simulink model "seven_segment_display"  (R2023b)
settings: Solver=VariableStepAuto  StartTime=0.0  StopTime=inf  RelTol=1e-3
libraries: simulink_extras x33
settings Model: ModifiedByFormat=ayber  Creator=ayber  LastModifiedBy=ayber
settings OptimizationCC: ReuseModelBlockBuffer=off

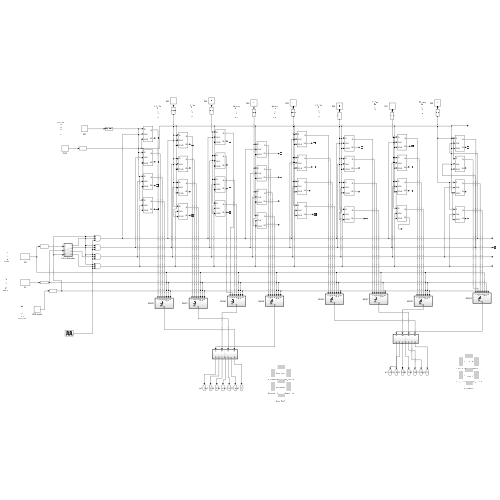
[thumbnail: Simulink's stored preview of the top-level diagram]
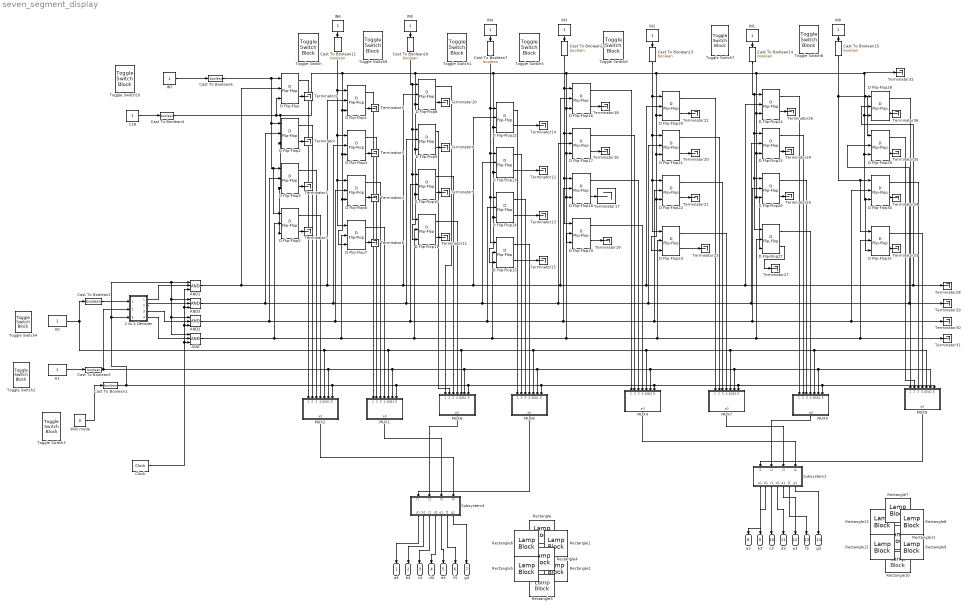
== system seven_segment_display ==
  2 to 4 Decoder : Subsystem  TreatAsAtomicUnit=on
  A0 : Constant
  A1 : Constant
  AND{,1..3} (4 alike) : Logic  Inputs=3  IconShape=distinctive  AllPortsSameDT=off  OutDataTypeStr=boolean
  CLR : Constant
  Cast To Boolean{1..2,4..7,10..15} (12 alike) : DataTypeConversion  OutDataTypeStr=boolean  SaturateOnIntegerOverflow=off  RndMeth=Floor
  Clock : simulink_extras/Flip Flops/Clock  period=2
  D Flip-Flop{,1..31} (32 alike) : simulink_extras/Flip Flops/D Flip-Flop
  IN{0..7} (8 alike) : Constant
  MUX1 : Subsystem  TreatAsAtomicUnit=on
  MUX2 : Subsystem  TreatAsAtomicUnit=on
  MUX4 : Subsystem  TreatAsAtomicUnit=on
  MUX5 : Subsystem  TreatAsAtomicUnit=on
  MUX6 : Subsystem  TreatAsAtomicUnit=on
  MUX7 : Subsystem  TreatAsAtomicUnit=on
  MUX8 : Subsystem  TreatAsAtomicUnit=on
  MUX9 : Subsystem  TreatAsAtomicUnit=on
  Rectangle{,1..13} (14 alike) : LampBlock  LabelPosition=Bottom  Icon=Rectangle
  Subsystem1 : Subsystem  TreatAsAtomicUnit=on
  Subsystem4 : Subsystem  TreatAsAtomicUnit=on
  Terminator{,1..36} (37 alike) : Terminator
  Toggle Switch{,1,5..10} (8 alike) : ToggleSwitchBlock
      settings: Values={{'Off', 'On'}, [0 1]}
  Toggle Switch2 : ToggleSwitchBlock  LabelPosition=Bottom
      settings: Values={{'Off', 'On'}, [0 1]}
  Toggle Switch3 : ToggleSwitchBlock  LabelPosition=Bottom
      settings: Values={{'Off', 'On'}, [0 1]}
  Toggle Switch4 : ToggleSwitchBlock  LabelPosition=Bottom
      settings: Values={{'Off', 'On'}, [0 1]}
  W/R mode : Constant  Value=0
  a4 : Outport
  b4 : Outport  Port=2
  c4 : Outport  Port=3
  d4 : Outport  Port=4
  e4 : Outport  Port=5
  f4 : Outport  Port=6
  g4 : Outport  Port=7
  a3 : Outport  Port=8
  b3 : Outport  Port=9
  c3 : Outport  Port=10
  d3 : Outport  Port=11
  e3 : Outport  Port=12
  f3 : Outport  Port=13
  g3 : Outport  Port=14
  wires:
  D Flip-Flop2/2 -> Terminator/1
  D Flip-Flop3/2 -> Terminator1/1
  CLR/1 -> Cast To Boolean4/1
  W/R mode/1 -> Cast To Boolean1/1
  A0/1 -> MUX9/5(A0), MUX5/5(A0), MUX7/5(A0), MUX4/5(A0), MUX8/5(A0), MUX6/5(A0), MUX1/5(A0), MUX2/5(A0), Cast To Boolean2/1
  A1/1 -> Cast To Boolean5/1
  D Flip-Flop/2 -> Terminator2/1
  D Flip-Flop5/2 -> Terminator7/1
  D Flip-Flop1/2 -> Terminator5/1
  D Flip-Flop7/2 -> Terminator6/1
  D Flip-Flop6/2 -> Terminator4/1
  D Flip-Flop4/2 -> Terminator3/1
  D Flip-Flop8/2 -> Terminator10/1
  D Flip-Flop11/2 -> Terminator11/1
  D Flip-Flop10/2 -> Terminator9/1
  D Flip-Flop9/2 -> Terminator8/1
  D Flip-Flop12/2 -> Terminator14/1
  D Flip-Flop15/2 -> Terminator15/1
  D Flip-Flop14/2 -> Terminator13/1
  D Flip-Flop13/2 -> Terminator12/1
  D Flip-Flop19/2 -> Terminator19/1
  D Flip-Flop18/2 -> Terminator17/1
  D Flip-Flop17/2 -> Terminator16/1
  D Flip-Flop16/2 -> Terminator18/1
  D Flip-Flop23/2 -> Terminator23/1
  D Flip-Flop22/2 -> Terminator21/1
  D Flip-Flop21/2 -> Terminator20/1
  D Flip-Flop20/2 -> Terminator22/1
  IN7/1 -> Cast To Boolean6/1
  Cast To Boolean6/1 -> D Flip-Flop/1, D Flip-Flop5/1, D Flip-Flop3/1, D Flip-Flop2/1
  IN4/1 -> Cast To Boolean7/1
  Cast To Boolean7/1 -> D Flip-Flop15/1, D Flip-Flop14/1, D Flip-Flop13/1, D Flip-Flop12/1
  IN5/1 -> Cast To Boolean10/1
  Cast To Boolean10/1 -> D Flip-Flop9/1, D Flip-Flop11/1, D Flip-Flop10/1, D Flip-Flop8/1
  IN6/1 -> Cast To Boolean11/1
  IN3/1 -> Cast To Boolean12/1
  IN2/1 -> Cast To Boolean13/1
  IN1/1 -> Cast To Boolean14/1
  D Flip-Flop24/2 -> Terminator26/1
  D Flip-Flop26/2 -> Terminator25/1
  D Flip-Flop27/2 -> Terminator27/1
  D Flip-Flop25/2 -> Terminator24/1
  Cast To Boolean14/1 -> D Flip-Flop27/1, D Flip-Flop26/1, D Flip-Flop25/1, D Flip-Flop24/1
  Cast To Boolean13/1 -> D Flip-Flop22/1, D Flip-Flop23/1, D Flip-Flop21/1, D Flip-Flop20/1
  Cast To Boolean12/1 -> D Flip-Flop19/1, D Flip-Flop18/1, D Flip-Flop17/1, D Flip-Flop16/1
  Cast To Boolean11/1 -> D Flip-Flop4/1, D Flip-Flop6/1, D Flip-Flop7/1, D Flip-Flop1/1
  Cast To Boolean5/1 -> MUX2/6(A1), MUX1/6(A1), MUX6/6(A1), MUX8/6(A1), MUX4/6(A1), MUX7/6(A1), MUX5/6(A1), MUX9/6(A1), 2 to 4 Decoder/2(In2)
  Cast To Boolean2/1 -> 2 to 4 Decoder/1(In1)
  Clock/1 -> AND1/3, AND3/3, AND2/3, AND/3
  Cast To Boolean1/1 -> MUX9/7(E), MUX5/7(E), MUX7/7(E), MUX4/7(E), MUX8/7(E), MUX6/7(E), MUX1/7(E), MUX2/7(E), AND/1, AND2/1, AND3/1, AND1/1, 2 to 4 Decoder/3(E)
  2 to 4 Decoder/1(Out1) -> AND1/2
  2 to 4 Decoder/2(Out2) -> AND3/2
  2 to 4 Decoder/3(Out3) -> AND2/2
  2 to 4 Decoder/4(Out4) -> AND/2
  AND1/1 -> Terminator28/1, D Flip-Flop28/2, D Flip-Flop24/2, D Flip-Flop20/2, D Flip-Flop16/2, D Flip-Flop12/2, D Flip-Flop8/2, D Flip-Flop1/2, D Flip-Flop/2
  AND2/1 -> Terminator30/1, D Flip-Flop30/2, D Flip-Flop26/2, D Flip-Flop22/2, D Flip-Flop18/2, D Flip-Flop14/2, D Flip-Flop10/2, D Flip-Flop6/2, D Flip-Flop3/2
  AND3/1 -> D Flip-Flop29/2, Terminator29/1, D Flip-Flop25/2, D Flip-Flop21/2, D Flip-Flop17/2, D Flip-Flop13/2, D Flip-Flop9/2, D Flip-Flop4/2, D Flip-Flop2/2
  AND/1 -> Terminator31/1, D Flip-Flop31/2, D Flip-Flop27/2, D Flip-Flop23/2, D Flip-Flop19/2, D Flip-Flop15/2, D Flip-Flop11/2, D Flip-Flop7/2, D Flip-Flop5/2
  Cast To Boolean4/1 -> D Flip-Flop1/3, D Flip-Flop4/3, D Flip-Flop6/3, D Flip-Flop7/3, D Flip-Flop31/3, D Flip-Flop30/3, D Flip-Flop29/3, D Flip-Flop28/3, Terminator32/1, D Flip-Flop27/3, D Flip-Flop26/3, D Flip-Flop25/3, D Flip-Flop24/3, D Flip-Flop23/3, D Flip-Flop22/3, D Flip-Flop21/3, D Flip-Flop20/3, D Flip-Flop19/3, D Flip-Flop18/3, D Flip-Flop17/3, D Flip-Flop16/3, D Flip-Flop15/3, D Flip-Flop14/3, D Flip-Flop13/3, D Flip-Flop12/3, D Flip-Flop8/3, D Flip-Flop9/3, D Flip-Flop10/3, D Flip-Flop11/3, D Flip-Flop5/3, D Flip-Flop3/3, D Flip-Flop2/3, D Flip-Flop/3
  D Flip-Flop5/1 -> MUX2/4(In6)
  D Flip-Flop7/1 -> MUX1/4(In6)
  D Flip-Flop15/1 -> MUX8/4(In6)
  D Flip-Flop19/1 -> MUX4/4(In6)
  D Flip-Flop23/1 -> MUX7/4(In6)
  D Flip-Flop27/1 -> MUX5/4(In6)
  D Flip-Flop26/1 -> MUX5/3(In5)
  D Flip-Flop22/1 -> MUX7/3(In5)
  D Flip-Flop25/1 -> MUX5/2(In4)
  D Flip-Flop24/1 -> MUX5/1(In3)
  D Flip-Flop21/1 -> MUX7/2(In4)
  D Flip-Flop20/1 -> MUX7/1(In3)
  D Flip-Flop18/1 -> MUX4/3(In5)
  D Flip-Flop17/1 -> MUX4/2(In4)
  D Flip-Flop16/1 -> MUX4/1(In3)
  D Flip-Flop3/1 -> MUX2/3(In5)
  D Flip-Flop/1 -> MUX2/1(In3)
  D Flip-Flop2/1 -> MUX2/2(In4)
  D Flip-Flop1/1 -> MUX1/1(In3)
  D Flip-Flop4/1 -> MUX1/2(In4)
  D Flip-Flop6/1 -> MUX1/3(In5)
  D Flip-Flop8/1 -> MUX6/1(In3)
  D Flip-Flop9/1 -> MUX6/2(In4)
  D Flip-Flop10/1 -> MUX6/3(In5)
  D Flip-Flop11/1 -> MUX6/4(In6)
  D Flip-Flop12/1 -> MUX8/1(In3)
  D Flip-Flop13/1 -> MUX8/2(In4)
  D Flip-Flop14/1 -> MUX8/3(In5)
  D Flip-Flop31/2 -> Terminator33/1
  D Flip-Flop30/2 -> Terminator34/1
  D Flip-Flop29/2 -> Terminator35/1
  D Flip-Flop28/2 -> Terminator36/1
  D Flip-Flop28/1 -> MUX9/1(In3)
  D Flip-Flop29/1 -> MUX9/2(In4)
  D Flip-Flop30/1 -> MUX9/3(In5)
  D Flip-Flop31/1 -> MUX9/4(In6)
  IN0/1 -> Cast To Boolean15/1
  Cast To Boolean15/1 -> D Flip-Flop29/1, D Flip-Flop28/1, D Flip-Flop31/1, D Flip-Flop30/1
  Subsystem4/1(a1) -> a4/1
  Subsystem4/4(d1) -> d4/1
  Subsystem4/5(e1) -> e4/1
  Subsystem4/7(g1) -> g4/1
  Subsystem4/6(f1) -> f4/1
  Subsystem4/3(c1) -> c4/1
  Subsystem4/2(b1) -> b4/1
  MUX2/1(a0) -> Subsystem4/4(I4)
  MUX1/1(a0) -> Subsystem4/3(I3)
  MUX6/1(a0) -> Subsystem4/2(I2)
  MUX8/1(a0) -> Subsystem4/1(I1)
  Subsystem1/5(e1) -> e3/1
  Subsystem1/4(d1) -> d3/1
  Subsystem1/6(f1) -> f3/1
  Subsystem1/1(a1) -> a3/1
  Subsystem1/2(b1) -> b3/1
  Subsystem1/7(g1) -> g3/1
  Subsystem1/3(c1) -> c3/1
  MUX4/1(a0) -> Subsystem1/4(I4)
  MUX7/1(a0) -> Subsystem1/3(I3)
  MUX5/1(a0) -> Subsystem1/2(I2)
  MUX9/1(a0) -> Subsystem1/1(I1)

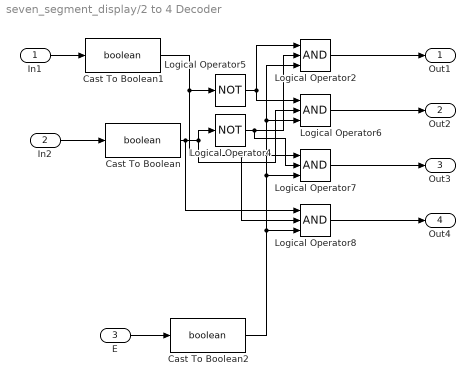
== system seven_segment_display/2 to 4 Decoder ==
  In1 : Inport
  In2 : Inport  Port=2
  E : Inport  Port=3
  Cast To Boolean : DataTypeConversion  OutDataTypeStr=boolean  SaturateOnIntegerOverflow=off  RndMeth=Floor
  Cast To Boolean1 : DataTypeConversion  OutDataTypeStr=boolean  SaturateOnIntegerOverflow=off  RndMeth=Floor
  Cast To Boolean2 : DataTypeConversion  OutDataTypeStr=boolean  SaturateOnIntegerOverflow=off  RndMeth=Floor
  Logical Operator{2,6..8} (4 alike) : Logic  Inputs=3  AllPortsSameDT=off  OutDataTypeStr=boolean
  Logical Operator4 : Logic  Operator=NOT  AllPortsSameDT=off  OutDataTypeStr=boolean
  Logical Operator5 : Logic  Operator=NOT  AllPortsSameDT=off  OutDataTypeStr=boolean
  Out1 : Outport
  Out2 : Outport  Port=2
  Out3 : Outport  Port=3
  Out4 : Outport  Port=4
  wires:
  Logical Operator8/1 -> Out4/1
  Logical Operator6/1 -> Out2/1
  Logical Operator2/1 -> Out1/1
  In1/1 -> Cast To Boolean1/1
  Cast To Boolean2/1 -> Logical Operator8/3, Logical Operator7/3, Logical Operator6/3, Logical Operator2/3
  Cast To Boolean/1 -> Logical Operator8/1, Logical Operator6/2, Logical Operator4/1
  Logical Operator7/1 -> Out3/1
  In2/1 -> Cast To Boolean/1
  Cast To Boolean1/1 -> Logical Operator8/2, Logical Operator7/1, Logical Operator5/1
  E/1 -> Cast To Boolean2/1
  Logical Operator5/1 -> Logical Operator6/1, Logical Operator2/1
  Logical Operator4/1 -> Logical Operator7/2, Logical Operator2/2

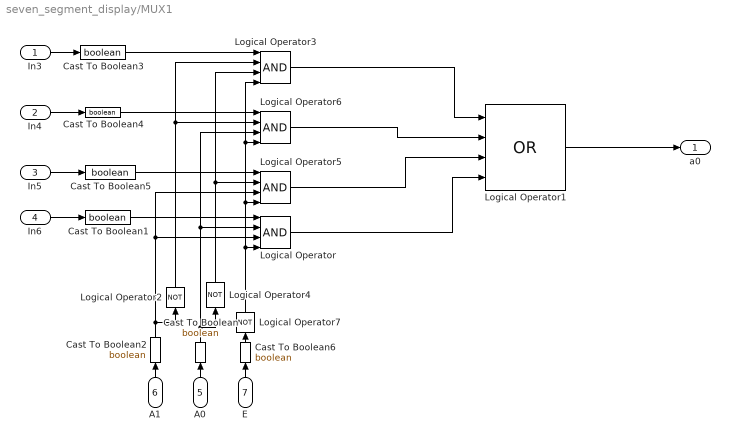
== system seven_segment_display/MUX1 ==
  In3 : Inport
  In4 : Inport  Port=2
  In5 : Inport  Port=3
  In6 : Inport  Port=4
  A0 : Inport  Port=5
  A1 : Inport  Port=6
  E : Inport  Port=7
  Cast To Boolean{,1..6} (7 alike) : DataTypeConversion  OutDataTypeStr=boolean  SaturateOnIntegerOverflow=off  RndMeth=Floor
  Logical Operator{,3,5..6} (4 alike) : Logic  Inputs=4  AllPortsSameDT=off  OutDataTypeStr=boolean
  Logical Operator1 : Logic  Operator=OR  Inputs=4  AllPortsSameDT=off  OutDataTypeStr=boolean
  Logical Operator2 : Logic  Operator=NOT  AllPortsSameDT=off  OutDataTypeStr=boolean
  Logical Operator4 : Logic  Operator=NOT  AllPortsSameDT=off  OutDataTypeStr=boolean
  Logical Operator7 : Logic  Operator=NOT  AllPortsSameDT=off  OutDataTypeStr=boolean
  a0 : Outport
  wires:
  A0/1 -> Cast To Boolean/1
  Logical Operator5/1 -> Logical Operator1/3
  In4/1 -> Cast To Boolean4/1
  Cast To Boolean3/1 -> Logical Operator3/1
  In5/1 -> Cast To Boolean5/1
  Cast To Boolean5/1 -> Logical Operator5/1
  Logical Operator1/1 -> a0/1
  Cast To Boolean1/1 -> Logical Operator/1
  Cast To Boolean4/1 -> Logical Operator6/1
  Logical Operator/1 -> Logical Operator1/4
  Logical Operator4/1 -> Logical Operator5/2, Logical Operator3/3
  In3/1 -> Cast To Boolean3/1
  Cast To Boolean/1 -> Logical Operator/2, Logical Operator6/3, Logical Operator4/1
  Logical Operator2/1 -> Logical Operator6/2, Logical Operator3/2
  A1/1 -> Cast To Boolean2/1
  In6/1 -> Cast To Boolean1/1
  Cast To Boolean2/1 -> Logical Operator/3, Logical Operator5/3, Logical Operator2/1
  Cast To Boolean6/1 -> Logical Operator7/1
  E/1 -> Cast To Boolean6/1
  Logical Operator7/1 -> Logical Operator3/4, Logical Operator6/4, Logical Operator5/4, Logical Operator/4
  Logical Operator6/1 -> Logical Operator1/2
  Logical Operator3/1 -> Logical Operator1/1

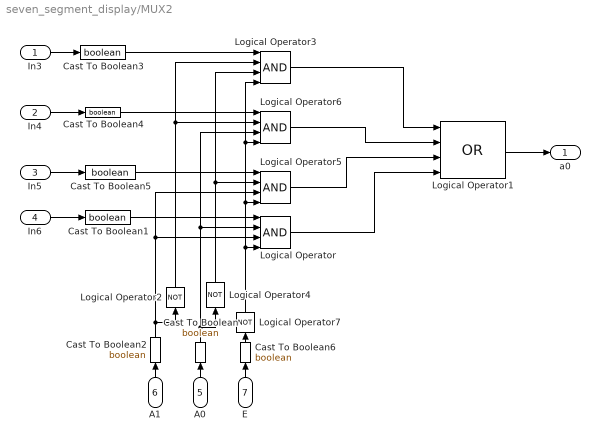
== system seven_segment_display/MUX2 ==
  In3 : Inport
  In4 : Inport  Port=2
  In5 : Inport  Port=3
  In6 : Inport  Port=4
  A0 : Inport  Port=5
  A1 : Inport  Port=6
  E : Inport  Port=7
  Cast To Boolean{,1..6} (7 alike) : DataTypeConversion  OutDataTypeStr=boolean  SaturateOnIntegerOverflow=off  RndMeth=Floor
  Logical Operator{,3,5..6} (4 alike) : Logic  Inputs=4  AllPortsSameDT=off  OutDataTypeStr=boolean
  Logical Operator1 : Logic  Operator=OR  Inputs=4  AllPortsSameDT=off  OutDataTypeStr=boolean
  Logical Operator2 : Logic  Operator=NOT  AllPortsSameDT=off  OutDataTypeStr=boolean
  Logical Operator4 : Logic  Operator=NOT  AllPortsSameDT=off  OutDataTypeStr=boolean
  Logical Operator7 : Logic  Operator=NOT  AllPortsSameDT=off  OutDataTypeStr=boolean
  a0 : Outport
  wires:
  A0/1 -> Cast To Boolean/1
  Logical Operator5/1 -> Logical Operator1/3
  In4/1 -> Cast To Boolean4/1
  Cast To Boolean3/1 -> Logical Operator3/1
  In5/1 -> Cast To Boolean5/1
  Cast To Boolean5/1 -> Logical Operator5/1
  Logical Operator1/1 -> a0/1
  Cast To Boolean1/1 -> Logical Operator/1
  Cast To Boolean4/1 -> Logical Operator6/1
  Logical Operator/1 -> Logical Operator1/4
  Logical Operator4/1 -> Logical Operator5/2, Logical Operator3/3
  In3/1 -> Cast To Boolean3/1
  Cast To Boolean/1 -> Logical Operator/2, Logical Operator6/3, Logical Operator4/1
  Logical Operator2/1 -> Logical Operator6/2, Logical Operator3/2
  A1/1 -> Cast To Boolean2/1
  In6/1 -> Cast To Boolean1/1
  Cast To Boolean2/1 -> Logical Operator/3, Logical Operator5/3, Logical Operator2/1
  Cast To Boolean6/1 -> Logical Operator7/1
  E/1 -> Cast To Boolean6/1
  Logical Operator7/1 -> Logical Operator3/4, Logical Operator6/4, Logical Operator5/4, Logical Operator/4
  Logical Operator6/1 -> Logical Operator1/2
  Logical Operator3/1 -> Logical Operator1/1

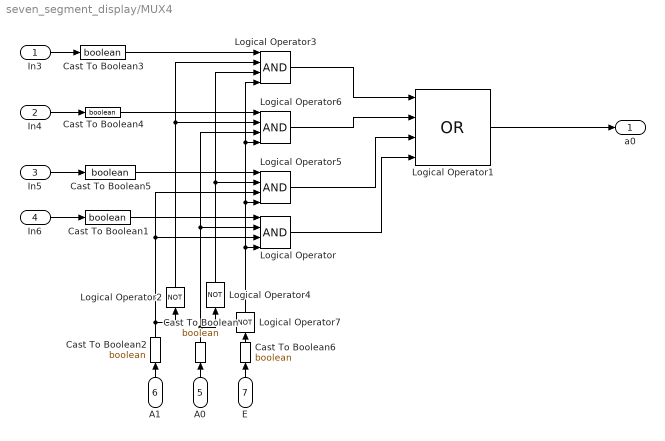
== system seven_segment_display/MUX4 ==
  In3 : Inport
  In4 : Inport  Port=2
  In5 : Inport  Port=3
  In6 : Inport  Port=4
  A0 : Inport  Port=5
  A1 : Inport  Port=6
  E : Inport  Port=7
  Cast To Boolean{,1..6} (7 alike) : DataTypeConversion  OutDataTypeStr=boolean  SaturateOnIntegerOverflow=off  RndMeth=Floor
  Logical Operator{,3,5..6} (4 alike) : Logic  Inputs=4  AllPortsSameDT=off  OutDataTypeStr=boolean
  Logical Operator1 : Logic  Operator=OR  Inputs=4  AllPortsSameDT=off  OutDataTypeStr=boolean
  Logical Operator2 : Logic  Operator=NOT  AllPortsSameDT=off  OutDataTypeStr=boolean
  Logical Operator4 : Logic  Operator=NOT  AllPortsSameDT=off  OutDataTypeStr=boolean
  Logical Operator7 : Logic  Operator=NOT  AllPortsSameDT=off  OutDataTypeStr=boolean
  a0 : Outport
  wires:
  A0/1 -> Cast To Boolean/1
  Logical Operator5/1 -> Logical Operator1/3
  In4/1 -> Cast To Boolean4/1
  Cast To Boolean3/1 -> Logical Operator3/1
  In5/1 -> Cast To Boolean5/1
  Cast To Boolean5/1 -> Logical Operator5/1
  Logical Operator1/1 -> a0/1
  Cast To Boolean1/1 -> Logical Operator/1
  Cast To Boolean4/1 -> Logical Operator6/1
  Logical Operator/1 -> Logical Operator1/4
  Logical Operator4/1 -> Logical Operator5/2, Logical Operator3/3
  In3/1 -> Cast To Boolean3/1
  Cast To Boolean/1 -> Logical Operator/2, Logical Operator6/3, Logical Operator4/1
  Logical Operator2/1 -> Logical Operator6/2, Logical Operator3/2
  A1/1 -> Cast To Boolean2/1
  In6/1 -> Cast To Boolean1/1
  Cast To Boolean2/1 -> Logical Operator/3, Logical Operator5/3, Logical Operator2/1
  Cast To Boolean6/1 -> Logical Operator7/1
  E/1 -> Cast To Boolean6/1
  Logical Operator7/1 -> Logical Operator3/4, Logical Operator6/4, Logical Operator5/4, Logical Operator/4
  Logical Operator3/1 -> Logical Operator1/1
  Logical Operator6/1 -> Logical Operator1/2

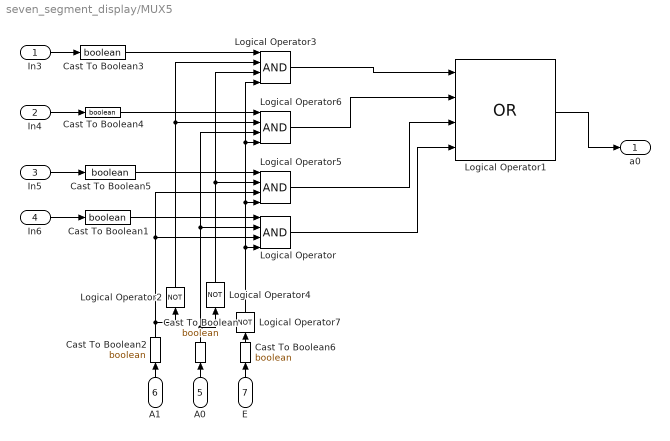
== system seven_segment_display/MUX5 ==
  In3 : Inport
  In4 : Inport  Port=2
  In5 : Inport  Port=3
  In6 : Inport  Port=4
  A0 : Inport  Port=5
  A1 : Inport  Port=6
  E : Inport  Port=7
  Cast To Boolean{,1..6} (7 alike) : DataTypeConversion  OutDataTypeStr=boolean  SaturateOnIntegerOverflow=off  RndMeth=Floor
  Logical Operator{,3,5..6} (4 alike) : Logic  Inputs=4  AllPortsSameDT=off  OutDataTypeStr=boolean
  Logical Operator1 : Logic  Operator=OR  Inputs=4  AllPortsSameDT=off  OutDataTypeStr=boolean
  Logical Operator2 : Logic  Operator=NOT  AllPortsSameDT=off  OutDataTypeStr=boolean
  Logical Operator4 : Logic  Operator=NOT  AllPortsSameDT=off  OutDataTypeStr=boolean
  Logical Operator7 : Logic  Operator=NOT  AllPortsSameDT=off  OutDataTypeStr=boolean
  a0 : Outport
  wires:
  A0/1 -> Cast To Boolean/1
  Logical Operator5/1 -> Logical Operator1/3
  In4/1 -> Cast To Boolean4/1
  Cast To Boolean3/1 -> Logical Operator3/1
  In5/1 -> Cast To Boolean5/1
  Cast To Boolean5/1 -> Logical Operator5/1
  Logical Operator1/1 -> a0/1
  Cast To Boolean1/1 -> Logical Operator/1
  Cast To Boolean4/1 -> Logical Operator6/1
  Logical Operator/1 -> Logical Operator1/4
  Logical Operator4/1 -> Logical Operator5/2, Logical Operator3/3
  In3/1 -> Cast To Boolean3/1
  Cast To Boolean/1 -> Logical Operator/2, Logical Operator6/3, Logical Operator4/1
  Logical Operator2/1 -> Logical Operator6/2, Logical Operator3/2
  A1/1 -> Cast To Boolean2/1
  In6/1 -> Cast To Boolean1/1
  Cast To Boolean2/1 -> Logical Operator/3, Logical Operator5/3, Logical Operator2/1
  Cast To Boolean6/1 -> Logical Operator7/1
  E/1 -> Cast To Boolean6/1
  Logical Operator7/1 -> Logical Operator3/4, Logical Operator6/4, Logical Operator5/4, Logical Operator/4
  Logical Operator6/1 -> Logical Operator1/2
  Logical Operator3/1 -> Logical Operator1/1

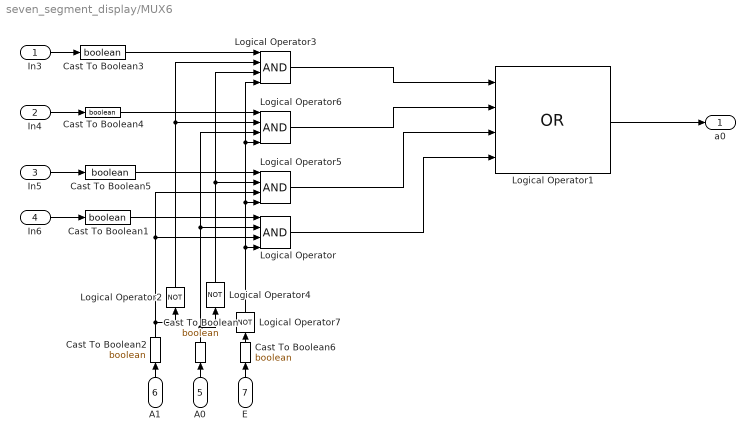
== system seven_segment_display/MUX6 ==
  In3 : Inport
  In4 : Inport  Port=2
  In5 : Inport  Port=3
  In6 : Inport  Port=4
  A0 : Inport  Port=5
  A1 : Inport  Port=6
  E : Inport  Port=7
  Cast To Boolean{,1..6} (7 alike) : DataTypeConversion  OutDataTypeStr=boolean  SaturateOnIntegerOverflow=off  RndMeth=Floor
  Logical Operator{,3,5..6} (4 alike) : Logic  Inputs=4  AllPortsSameDT=off  OutDataTypeStr=boolean
  Logical Operator1 : Logic  Operator=OR  Inputs=4  AllPortsSameDT=off  OutDataTypeStr=boolean
  Logical Operator2 : Logic  Operator=NOT  AllPortsSameDT=off  OutDataTypeStr=boolean
  Logical Operator4 : Logic  Operator=NOT  AllPortsSameDT=off  OutDataTypeStr=boolean
  Logical Operator7 : Logic  Operator=NOT  AllPortsSameDT=off  OutDataTypeStr=boolean
  a0 : Outport
  wires:
  A0/1 -> Cast To Boolean/1
  Logical Operator5/1 -> Logical Operator1/3
  In4/1 -> Cast To Boolean4/1
  Cast To Boolean3/1 -> Logical Operator3/1
  In5/1 -> Cast To Boolean5/1
  Cast To Boolean5/1 -> Logical Operator5/1
  Logical Operator1/1 -> a0/1
  Cast To Boolean1/1 -> Logical Operator/1
  Cast To Boolean4/1 -> Logical Operator6/1
  Logical Operator/1 -> Logical Operator1/4
  Logical Operator4/1 -> Logical Operator5/2, Logical Operator3/3
  In3/1 -> Cast To Boolean3/1
  Cast To Boolean/1 -> Logical Operator/2, Logical Operator6/3, Logical Operator4/1
  Logical Operator2/1 -> Logical Operator6/2, Logical Operator3/2
  A1/1 -> Cast To Boolean2/1
  In6/1 -> Cast To Boolean1/1
  Cast To Boolean2/1 -> Logical Operator/3, Logical Operator5/3, Logical Operator2/1
  Cast To Boolean6/1 -> Logical Operator7/1
  E/1 -> Cast To Boolean6/1
  Logical Operator7/1 -> Logical Operator3/4, Logical Operator6/4, Logical Operator5/4, Logical Operator/4
  Logical Operator3/1 -> Logical Operator1/1
  Logical Operator6/1 -> Logical Operator1/2

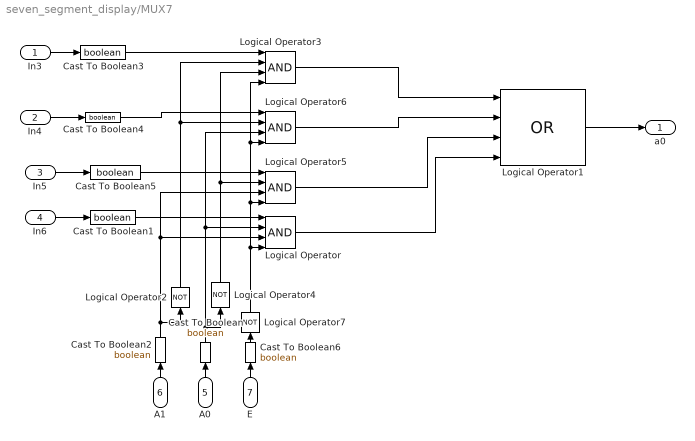
== system seven_segment_display/MUX7 ==
  In3 : Inport
  In4 : Inport  Port=2
  In5 : Inport  Port=3
  In6 : Inport  Port=4
  A0 : Inport  Port=5
  A1 : Inport  Port=6
  E : Inport  Port=7
  Cast To Boolean{,1..6} (7 alike) : DataTypeConversion  OutDataTypeStr=boolean  SaturateOnIntegerOverflow=off  RndMeth=Floor
  Logical Operator{,3,5..6} (4 alike) : Logic  Inputs=4  AllPortsSameDT=off  OutDataTypeStr=boolean
  Logical Operator1 : Logic  Operator=OR  Inputs=4  AllPortsSameDT=off  OutDataTypeStr=boolean
  Logical Operator2 : Logic  Operator=NOT  AllPortsSameDT=off  OutDataTypeStr=boolean
  Logical Operator4 : Logic  Operator=NOT  AllPortsSameDT=off  OutDataTypeStr=boolean
  Logical Operator7 : Logic  Operator=NOT  AllPortsSameDT=off  OutDataTypeStr=boolean
  a0 : Outport
  wires:
  A0/1 -> Cast To Boolean/1
  Logical Operator5/1 -> Logical Operator1/3
  In4/1 -> Cast To Boolean4/1
  Cast To Boolean3/1 -> Logical Operator3/1
  In5/1 -> Cast To Boolean5/1
  Cast To Boolean5/1 -> Logical Operator5/1
  Logical Operator1/1 -> a0/1
  Cast To Boolean1/1 -> Logical Operator/1
  Cast To Boolean4/1 -> Logical Operator6/1
  Logical Operator/1 -> Logical Operator1/4
  Logical Operator4/1 -> Logical Operator5/2, Logical Operator3/3
  In3/1 -> Cast To Boolean3/1
  Cast To Boolean/1 -> Logical Operator/2, Logical Operator6/3, Logical Operator4/1
  Logical Operator2/1 -> Logical Operator6/2, Logical Operator3/2
  A1/1 -> Cast To Boolean2/1
  In6/1 -> Cast To Boolean1/1
  Cast To Boolean2/1 -> Logical Operator/3, Logical Operator5/3, Logical Operator2/1
  Cast To Boolean6/1 -> Logical Operator7/1
  E/1 -> Cast To Boolean6/1
  Logical Operator7/1 -> Logical Operator3/4, Logical Operator6/4, Logical Operator5/4, Logical Operator/4
  Logical Operator6/1 -> Logical Operator1/2
  Logical Operator3/1 -> Logical Operator1/1

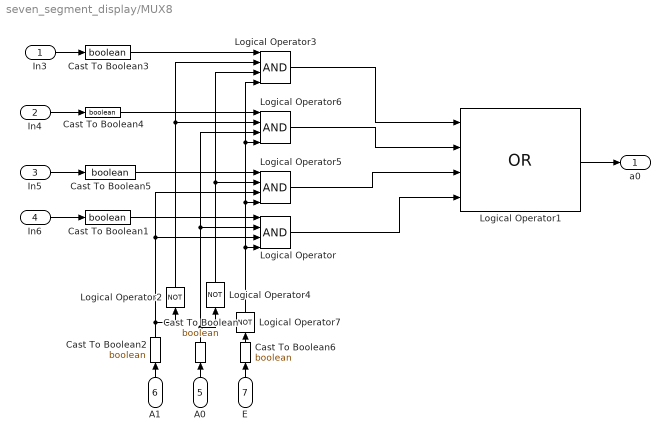
== system seven_segment_display/MUX8 ==
  In3 : Inport
  In4 : Inport  Port=2
  In5 : Inport  Port=3
  In6 : Inport  Port=4
  A0 : Inport  Port=5
  A1 : Inport  Port=6
  E : Inport  Port=7
  Cast To Boolean{,1..6} (7 alike) : DataTypeConversion  OutDataTypeStr=boolean  SaturateOnIntegerOverflow=off  RndMeth=Floor
  Logical Operator{,3,5..6} (4 alike) : Logic  Inputs=4  AllPortsSameDT=off  OutDataTypeStr=boolean
  Logical Operator1 : Logic  Operator=OR  Inputs=4  AllPortsSameDT=off  OutDataTypeStr=boolean
  Logical Operator2 : Logic  Operator=NOT  AllPortsSameDT=off  OutDataTypeStr=boolean
  Logical Operator4 : Logic  Operator=NOT  AllPortsSameDT=off  OutDataTypeStr=boolean
  Logical Operator7 : Logic  Operator=NOT  AllPortsSameDT=off  OutDataTypeStr=boolean
  a0 : Outport
  wires:
  A0/1 -> Cast To Boolean/1
  Logical Operator5/1 -> Logical Operator1/3
  In4/1 -> Cast To Boolean4/1
  Cast To Boolean3/1 -> Logical Operator3/1
  In5/1 -> Cast To Boolean5/1
  Cast To Boolean5/1 -> Logical Operator5/1
  Logical Operator1/1 -> a0/1
  Cast To Boolean1/1 -> Logical Operator/1
  Cast To Boolean4/1 -> Logical Operator6/1
  Logical Operator/1 -> Logical Operator1/4
  Logical Operator4/1 -> Logical Operator5/2, Logical Operator3/3
  In3/1 -> Cast To Boolean3/1
  Cast To Boolean/1 -> Logical Operator/2, Logical Operator6/3, Logical Operator4/1
  Logical Operator2/1 -> Logical Operator6/2, Logical Operator3/2
  A1/1 -> Cast To Boolean2/1
  In6/1 -> Cast To Boolean1/1
  Cast To Boolean2/1 -> Logical Operator/3, Logical Operator5/3, Logical Operator2/1
  Cast To Boolean6/1 -> Logical Operator7/1
  E/1 -> Cast To Boolean6/1
  Logical Operator7/1 -> Logical Operator3/4, Logical Operator6/4, Logical Operator5/4, Logical Operator/4
  Logical Operator3/1 -> Logical Operator1/1
  Logical Operator6/1 -> Logical Operator1/2

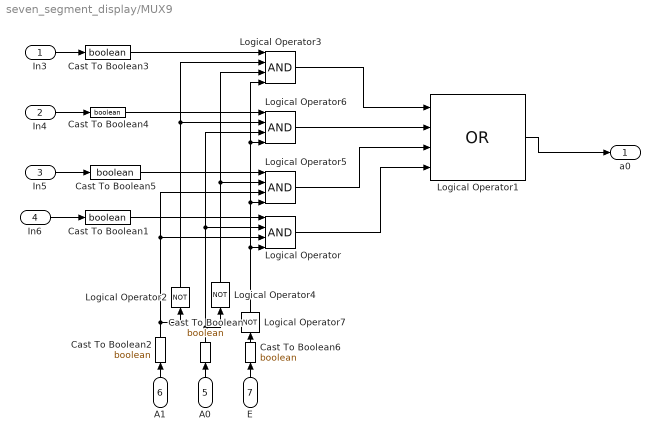
== system seven_segment_display/MUX9 ==
  In3 : Inport
  In4 : Inport  Port=2
  In5 : Inport  Port=3
  In6 : Inport  Port=4
  A0 : Inport  Port=5
  A1 : Inport  Port=6
  E : Inport  Port=7
  Cast To Boolean{,1..6} (7 alike) : DataTypeConversion  OutDataTypeStr=boolean  SaturateOnIntegerOverflow=off  RndMeth=Floor
  Logical Operator{,3,5..6} (4 alike) : Logic  Inputs=4  AllPortsSameDT=off  OutDataTypeStr=boolean
  Logical Operator1 : Logic  Operator=OR  Inputs=4  AllPortsSameDT=off  OutDataTypeStr=boolean
  Logical Operator2 : Logic  Operator=NOT  AllPortsSameDT=off  OutDataTypeStr=boolean
  Logical Operator4 : Logic  Operator=NOT  AllPortsSameDT=off  OutDataTypeStr=boolean
  Logical Operator7 : Logic  Operator=NOT  AllPortsSameDT=off  OutDataTypeStr=boolean
  a0 : Outport
  wires:
  A0/1 -> Cast To Boolean/1
  Logical Operator5/1 -> Logical Operator1/3
  In4/1 -> Cast To Boolean4/1
  Cast To Boolean3/1 -> Logical Operator3/1
  In5/1 -> Cast To Boolean5/1
  Cast To Boolean5/1 -> Logical Operator5/1
  Logical Operator1/1 -> a0/1
  Cast To Boolean1/1 -> Logical Operator/1
  Cast To Boolean4/1 -> Logical Operator6/1
  Logical Operator/1 -> Logical Operator1/4
  Logical Operator4/1 -> Logical Operator5/2, Logical Operator3/3
  In3/1 -> Cast To Boolean3/1
  Cast To Boolean/1 -> Logical Operator/2, Logical Operator6/3, Logical Operator4/1
  Logical Operator2/1 -> Logical Operator6/2, Logical Operator3/2
  A1/1 -> Cast To Boolean2/1
  In6/1 -> Cast To Boolean1/1
  Cast To Boolean2/1 -> Logical Operator/3, Logical Operator5/3, Logical Operator2/1
  Cast To Boolean6/1 -> Logical Operator7/1
  E/1 -> Cast To Boolean6/1
  Logical Operator7/1 -> Logical Operator3/4, Logical Operator6/4, Logical Operator5/4, Logical Operator/4
  Logical Operator3/1 -> Logical Operator1/1
  Logical Operator6/1 -> Logical Operator1/2

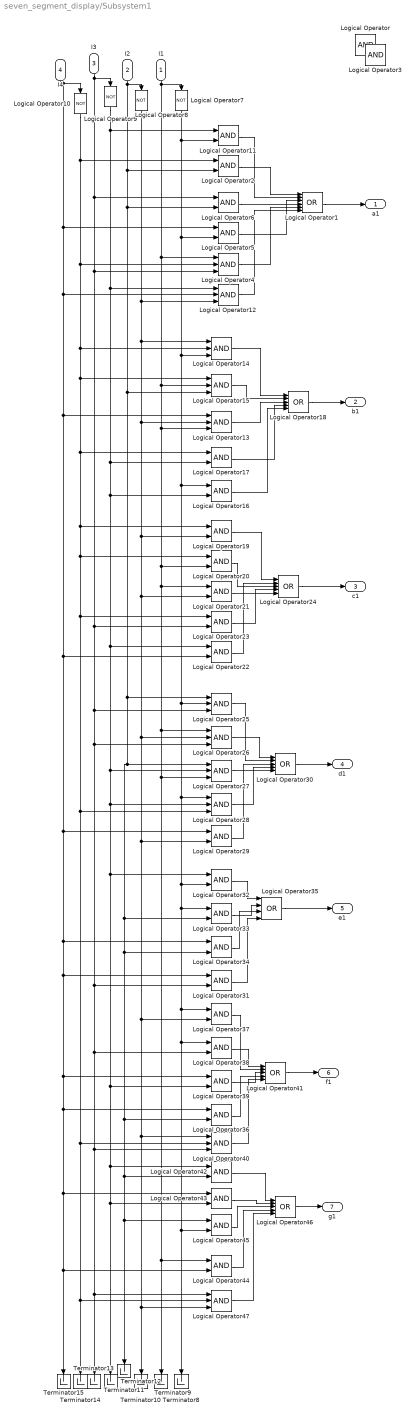
== system seven_segment_display/Subsystem1 ==
  I1 : Inport
  I2 : Inport  Port=2
  I3 : Inport  Port=3
  I4 : Inport  Port=4
  Logical Operator{,2..3,5..6,11,16..17,19..23,29,31..34,36..39,42..45} (26 alike) : Logic  AllPortsSameDT=off  OutDataTypeStr=boolean
  Logical Operator1 : Logic  Operator=OR  Inputs=6  AllPortsSameDT=off  OutDataTypeStr=boolean
  Logical Operator{7..10} (4 alike) : Logic  Operator=NOT  AllPortsSameDT=off  OutDataTypeStr=boolean
  Logical Operator{4,12..15,25..28,40,47} (11 alike) : Logic  Inputs=3  AllPortsSameDT=off  OutDataTypeStr=boolean
  Logical Operator{18,24,30,41,46} (5 alike) : Logic  Operator=OR  Inputs=5  AllPortsSameDT=off  OutDataTypeStr=boolean
  Logical Operator35 : Logic  Operator=OR  Inputs=4  AllPortsSameDT=off  OutDataTypeStr=boolean
  Terminator{8..15} (8 alike) : Terminator
  a1 : Outport
  b1 : Outport  Port=2
  c1 : Outport  Port=3
  d1 : Outport  Port=4
  e1 : Outport  Port=5
  f1 : Outport  Port=6
  g1 : Outport  Port=7
  wires:
  I1/1 -> Logical Operator7/1, Logical Operator4/1, Logical Operator26/1, Logical Operator27/3, Logical Operator44/1, Terminator9/1, Logical Operator21/1, Logical Operator20/2, Logical Operator13/3, Logical Operator15/2
  I4/1 -> Logical Operator5/1, Logical Operator12/2, Logical Operator29/1, Logical Operator31/1, Logical Operator39/1, Logical Operator43/1, Terminator15/1, Logical Operator44/2, Logical Operator36/1, Logical Operator34/1, Logical Operator22/2, Logical Operator13/1, Logical Operator10/1
  I3/1 -> Terminator13/1, Logical Operator47/1, Logical Operator40/3, Logical Operator38/2, Logical Operator31/2, Logical Operator26/3, Logical Operator25/3, Logical Operator23/2, Logical Operator4/3, Logical Operator6/1, Logical Operator9/1
  I2/1 -> Logical Operator15/3, Logical Operator33/2, Logical Operator45/1, Terminator11/1, Logical Operator42/2, Logical Operator36/2, Logical Operator34/2, Logical Operator27/1, Logical Operator25/1, Logical Operator6/2, Logical Operator2/2, Logical Operator8/1
  Logical Operator7/1 -> Logical Operator5/2, Logical Operator16/1, Logical Operator28/1, Logical Operator32/2, Logical Operator33/1, Logical Operator37/1, Logical Operator38/1, Terminator8/1, Logical Operator45/2, Logical Operator25/2, Logical Operator14/3, Logical Operator11/2
  Logical Operator8/1 -> Logical Operator14/1, Logical Operator21/2, Logical Operator26/2, Logical Operator40/1, Terminator10/1, Logical Operator47/3, Logical Operator37/2, Logical Operator29/2, Logical Operator19/2, Logical Operator13/2, Logical Operator12/3
  Logical Operator9/1 -> Logical Operator11/1, Logical Operator12/1, Logical Operator16/2, Logical Operator22/1, Logical Operator27/2, Logical Operator28/2, Terminator12/1, Logical Operator43/2, Logical Operator42/1, Logical Operator39/2, Logical Operator32/1, Logical Operator17/2
  Logical Operator10/1 -> Logical Operator2/1, Logical Operator4/2, Logical Operator14/2, Logical Operator15/1, Logical Operator28/3, Logical Operator40/2, Logical Operator47/2, Terminator14/1, Logical Operator23/1, Logical Operator20/1, Logical Operator19/1, Logical Operator17/1
  Logical Operator6/1 -> Logical Operator1/4
  Logical Operator4/1 -> Logical Operator1/5
  Logical Operator12/1 -> Logical Operator1/6
  Logical Operator5/1 -> Logical Operator1/3
  Logical Operator2/1 -> Logical Operator1/1
  Logical Operator11/1 -> Logical Operator1/2
  Logical Operator1/1 -> a1/1
  Logical Operator14/1 -> Logical Operator18/1
  Logical Operator15/1 -> Logical Operator18/2
  Logical Operator13/1 -> Logical Operator18/3
  Logical Operator17/1 -> Logical Operator18/4
  Logical Operator16/1 -> Logical Operator18/5
  Logical Operator18/1 -> b1/1
  Logical Operator21/1 -> Logical Operator24/5
  Logical Operator23/1 -> Logical Operator24/4
  Logical Operator22/1 -> Logical Operator24/2
  Logical Operator20/1 -> Logical Operator24/3
  Logical Operator19/1 -> Logical Operator24/1
  Logical Operator24/1 -> c1/1
  Logical Operator27/1 -> Logical Operator30/5
  Logical Operator28/1 -> Logical Operator30/4
  Logical Operator29/1 -> Logical Operator30/3
  Logical Operator26/1 -> Logical Operator30/1
  Logical Operator25/1 -> Logical Operator30/2
  Logical Operator30/1 -> d1/1
  Logical Operator31/1 -> Logical Operator35/4
  Logical Operator34/1 -> Logical Operator35/3
  Logical Operator33/1 -> Logical Operator35/2
  Logical Operator32/1 -> Logical Operator35/1
  Logical Operator35/1 -> e1/1
  Logical Operator40/1 -> Logical Operator41/5
  Logical Operator36/1 -> Logical Operator41/4
  Logical Operator39/1 -> Logical Operator41/3
  Logical Operator38/1 -> Logical Operator41/1
  Logical Operator37/1 -> Logical Operator41/2
  Logical Operator41/1 -> f1/1
  Logical Operator46/1 -> g1/1
  Logical Operator47/1 -> Logical Operator46/5
  Logical Operator44/1 -> Logical Operator46/4
  Logical Operator45/1 -> Logical Operator46/3
  Logical Operator43/1 -> Logical Operator46/2
  Logical Operator42/1 -> Logical Operator46/1

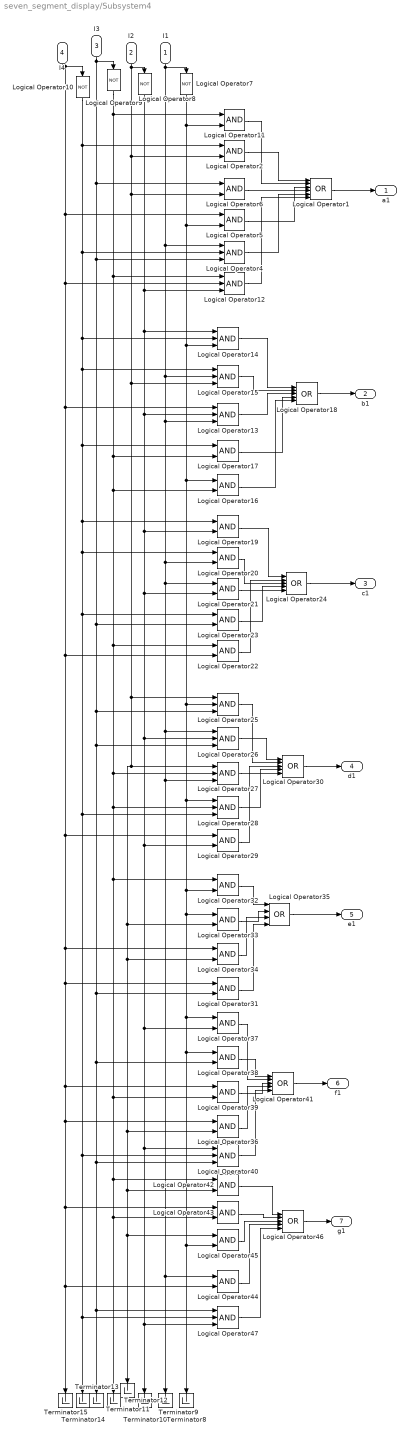
== system seven_segment_display/Subsystem4 ==
  I1 : Inport
  I2 : Inport  Port=2
  I3 : Inport  Port=3
  I4 : Inport  Port=4
  Logical Operator1 : Logic  Operator=OR  Inputs=6  AllPortsSameDT=off  OutDataTypeStr=boolean
  Logical Operator{7..10} (4 alike) : Logic  Operator=NOT  AllPortsSameDT=off  OutDataTypeStr=boolean
  Logical Operator{2,5..6,11,16..17,19..23,29,31..34,36..39,42..45} (24 alike) : Logic  AllPortsSameDT=off  OutDataTypeStr=boolean
  Logical Operator{4,12..15,25..28,40,47} (11 alike) : Logic  Inputs=3  AllPortsSameDT=off  OutDataTypeStr=boolean
  Logical Operator{18,24,30,41,46} (5 alike) : Logic  Operator=OR  Inputs=5  AllPortsSameDT=off  OutDataTypeStr=boolean
  Logical Operator35 : Logic  Operator=OR  Inputs=4  AllPortsSameDT=off  OutDataTypeStr=boolean
  Terminator{8..15} (8 alike) : Terminator
  a1 : Outport
  b1 : Outport  Port=2
  c1 : Outport  Port=3
  d1 : Outport  Port=4
  e1 : Outport  Port=5
  f1 : Outport  Port=6
  g1 : Outport  Port=7
  wires:
  I1/1 -> Logical Operator7/1, Logical Operator4/1, Logical Operator26/1, Logical Operator27/3, Logical Operator44/1, Terminator9/1, Logical Operator21/1, Logical Operator20/2, Logical Operator13/3, Logical Operator15/2
  I4/1 -> Logical Operator5/1, Logical Operator12/2, Logical Operator29/1, Logical Operator31/1, Logical Operator39/1, Logical Operator43/1, Terminator15/1, Logical Operator44/2, Logical Operator36/1, Logical Operator34/1, Logical Operator22/2, Logical Operator13/1, Logical Operator10/1
  I3/1 -> Terminator13/1, Logical Operator47/1, Logical Operator40/3, Logical Operator38/2, Logical Operator31/2, Logical Operator26/3, Logical Operator25/3, Logical Operator23/2, Logical Operator4/3, Logical Operator6/1, Logical Operator9/1
  I2/1 -> Logical Operator15/3, Logical Operator33/2, Logical Operator45/1, Terminator11/1, Logical Operator42/2, Logical Operator36/2, Logical Operator34/2, Logical Operator27/1, Logical Operator25/1, Logical Operator6/2, Logical Operator2/2, Logical Operator8/1
  Logical Operator7/1 -> Logical Operator5/2, Logical Operator16/1, Logical Operator28/1, Logical Operator32/2, Logical Operator33/1, Logical Operator37/1, Logical Operator38/1, Terminator8/1, Logical Operator45/2, Logical Operator25/2, Logical Operator14/3, Logical Operator11/2
  Logical Operator8/1 -> Logical Operator14/1, Logical Operator21/2, Logical Operator26/2, Logical Operator40/1, Terminator10/1, Logical Operator47/3, Logical Operator37/2, Logical Operator29/2, Logical Operator19/2, Logical Operator13/2, Logical Operator12/3
  Logical Operator9/1 -> Logical Operator11/1, Logical Operator12/1, Logical Operator16/2, Logical Operator22/1, Logical Operator27/2, Logical Operator28/2, Terminator12/1, Logical Operator43/2, Logical Operator42/1, Logical Operator39/2, Logical Operator32/1, Logical Operator17/2
  Logical Operator10/1 -> Logical Operator2/1, Logical Operator4/2, Logical Operator14/2, Logical Operator15/1, Logical Operator28/3, Logical Operator40/2, Logical Operator47/2, Terminator14/1, Logical Operator23/1, Logical Operator20/1, Logical Operator19/1, Logical Operator17/1
  Logical Operator6/1 -> Logical Operator1/4
  Logical Operator4/1 -> Logical Operator1/5
  Logical Operator12/1 -> Logical Operator1/6
  Logical Operator5/1 -> Logical Operator1/3
  Logical Operator2/1 -> Logical Operator1/1
  Logical Operator11/1 -> Logical Operator1/2
  Logical Operator1/1 -> a1/1
  Logical Operator14/1 -> Logical Operator18/1
  Logical Operator15/1 -> Logical Operator18/2
  Logical Operator13/1 -> Logical Operator18/3
  Logical Operator17/1 -> Logical Operator18/4
  Logical Operator16/1 -> Logical Operator18/5
  Logical Operator18/1 -> b1/1
  Logical Operator21/1 -> Logical Operator24/5
  Logical Operator23/1 -> Logical Operator24/4
  Logical Operator22/1 -> Logical Operator24/2
  Logical Operator20/1 -> Logical Operator24/3
  Logical Operator19/1 -> Logical Operator24/1
  Logical Operator24/1 -> c1/1
  Logical Operator27/1 -> Logical Operator30/5
  Logical Operator28/1 -> Logical Operator30/4
  Logical Operator29/1 -> Logical Operator30/3
  Logical Operator26/1 -> Logical Operator30/1
  Logical Operator25/1 -> Logical Operator30/2
  Logical Operator30/1 -> d1/1
  Logical Operator31/1 -> Logical Operator35/4
  Logical Operator34/1 -> Logical Operator35/3
  Logical Operator33/1 -> Logical Operator35/2
  Logical Operator32/1 -> Logical Operator35/1
  Logical Operator35/1 -> e1/1
  Logical Operator40/1 -> Logical Operator41/5
  Logical Operator36/1 -> Logical Operator41/4
  Logical Operator39/1 -> Logical Operator41/3
  Logical Operator38/1 -> Logical Operator41/1
  Logical Operator37/1 -> Logical Operator41/2
  Logical Operator41/1 -> f1/1
  Logical Operator46/1 -> g1/1
  Logical Operator47/1 -> Logical Operator46/5
  Logical Operator44/1 -> Logical Operator46/4
  Logical Operator45/1 -> Logical Operator46/3
  Logical Operator43/1 -> Logical Operator46/2
  Logical Operator42/1 -> Logical Operator46/1
